simulink model "lift"  (R2015b)
settings: Solver=FixedStepAuto  StartTime=0.0  StopTime=200  FixedStep=1  MaxStep=10  RelTol=1e-3
libraries: simulink x8
settings Model: Creator=DNikolaev  LastModifiedBy=DNikolaev

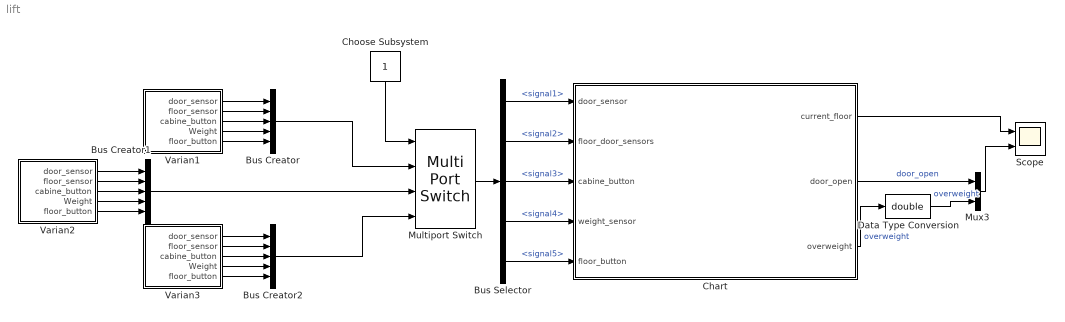
== system lift ==
  Bus Creator : BusCreator  Inputs=5
  Bus Creator1 : BusCreator  Inputs=5
  Bus Creator2 : BusCreator  Inputs=5
  Bus Selector : BusSelector  OutputSignals=signal1,signal2,signal3,signal4,signal5
  Chart : Stateflow chart  TreatAsAtomicUnit=on
  Choose Subsystem : Constant
  Data Type Conversion : DataTypeConversion  OutDataTypeStr=double
  Multiport Switch : MultiPortSwitch
  Mux3 : Mux  Inputs=2
  Scope : Scope  NumInputPorts=2
  Varian1 : Subsystem
  Varian2 : Subsystem
  Varian3 : Subsystem
  wires:
  Chart/1(current_floor) -> Scope/1
  Chart/2(door_open) -> Mux3/1  "door_open"
  Varian1/1(door_sensor) -> Bus Creator/1
  Varian1/2(floor_sensor) -> Bus Creator/2
  Varian1/3(cabine_button) -> Bus Creator/3
  Varian1/4(Weight) -> Bus Creator/4
  Varian1/5(floor_button) -> Bus Creator/5
  Multiport Switch/1 -> Bus Selector/1
  Bus Creator/1 -> Multiport Switch/2
  Bus Creator1/1 -> Multiport Switch/3
  Bus Creator2/1 -> Multiport Switch/4
  Choose Subsystem/1 -> Multiport Switch/1
  Varian3/1(door_sensor) -> Bus Creator2/1
  Varian3/2(floor_sensor) -> Bus Creator2/2
  Varian3/3(cabine_button) -> Bus Creator2/3
  Varian3/4(Weight) -> Bus Creator2/4
  Varian3/5(floor_button) -> Bus Creator2/5
  Chart/3(overweight) -> Data Type Conversion/1  "overweight"
  Mux3/1 -> Scope/2
  Varian2/3(cabine_button) -> Bus Creator1/3
  Varian2/2(floor_sensor) -> Bus Creator1/2
  Varian2/5(floor_button) -> Bus Creator1/5
  Varian2/4(Weight) -> Bus Creator1/4
  Varian2/1(door_sensor) -> Bus Creator1/1
  Bus Selector/5 -> Chart/5(floor_button)  "<signal5>"
  Bus Selector/4 -> Chart/4(weight_sensor)  "<signal4>"
  Bus Selector/2 -> Chart/2(floor_door_sensors)  "<signal2>"
  Bus Selector/1 -> Chart/1(door_sensor)  "<signal1>"
  Bus Selector/3 -> Chart/3(cabine_button)  "<signal3>"
  Data Type Conversion/1 -> Mux3/2  "overweight"

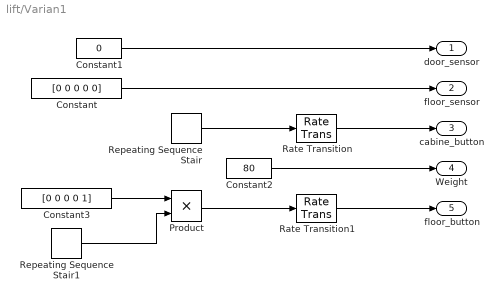
== system lift/Varian1 ==
  Constant : Constant  Value=[0 0 0 0 0]
  Constant1 : Constant  Value=0
  Constant2 : Constant  Value=80
  Constant3 : Constant  Value=[0 0 0 0 1]
  Product : Product
  Rate Transition : RateTransition  OutPortSampleTime=1
  Rate Transition1 : RateTransition  OutPortSampleTime=1
  Repeating Sequence Stair : simulink/Sources/Repeating Sequence Stair  OutValues=[0 0 0 0 0 0 0 0 0 2 0 0 0 0 0 0]  tsamp=10  OutMin=[]  OutMax=[]  OutDataTypeStr=double  OutputDataTypeScalingMode=double  OutDataType=fixdt(0,8)  ConRadixGroup=Best Precision: Vector-wise  OutScaling=2^-12
  Repeating Sequence Stair1 : simulink/Sources/Repeating Sequence Stair  OutValues=[0 0 1 0 0 0 0 0 0 0 0 0 0 0 0 0]  tsamp=10  OutMin=[]  OutMax=[]  OutDataTypeStr=double  OutputDataTypeScalingMode=double  OutDataType=fixdt(0,8)  ConRadixGroup=Best Precision: Vector-wise  OutScaling=2^-12
  door_sensor : Outport
  floor_sensor : Outport  Port=2
  cabine_button : Outport  Port=3
  Weight : Outport  Port=4
  floor_button : Outport  Port=5
  wires:
  Constant2/1 -> Weight/1
  Rate Transition/1 -> cabine_button/1
  Constant/1 -> floor_sensor/1
  Constant1/1 -> door_sensor/1
  Repeating Sequence Stair/1 -> Rate Transition/1
  Constant3/1 -> Product/1
  Rate Transition1/1 -> floor_button/1
  Repeating Sequence Stair1/1 -> Product/2
  Product/1 -> Rate Transition1/1

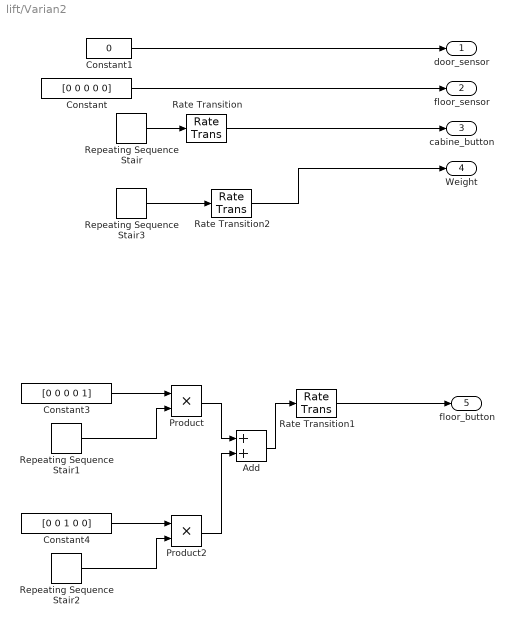
== system lift/Varian2 ==
  Add : Sum
  Constant : Constant  Value=[0 0 0 0 0]
  Constant1 : Constant  Value=0
  Constant3 : Constant  Value=[0 0 0 0 1]
  Constant4 : Constant  Value=[0 0 1 0 0]
  Product : Product
  Product2 : Product
  Rate Transition : RateTransition  OutPortSampleTime=1
  Rate Transition1 : RateTransition  OutPortSampleTime=1
  Rate Transition2 : RateTransition  OutPortSampleTime=1
  Repeating Sequence Stair : simulink/Sources/Repeating Sequence Stair  OutValues=[0 0 0 0 0 0 0 0 2 2 0 0 0 0 0 0]  tsamp=10  OutMin=[]  OutMax=[]  OutDataTypeStr=double  OutputDataTypeScalingMode=double  OutDataType=fixdt(0,8)  ConRadixGroup=Best Precision: Vector-wise  OutScaling=2^-12
  Repeating Sequence Stair1 : simulink/Sources/Repeating Sequence Stair  OutValues=[0 0 1 0 0 0 0 0 0 0 0 0 0 0 0 0]  tsamp=10  OutMin=[]  OutMax=[]  OutDataTypeStr=double  OutputDataTypeScalingMode=double  OutDataType=fixdt(0,8)  ConRadixGroup=Best Precision: Vector-wise  OutScaling=2^-12
  Repeating Sequence Stair2 : simulink/Sources/Repeating Sequence Stair  OutValues=[0 0 0 0 0 0 0 0 0 0 0 0 0 1 0]  tsamp=10  OutMin=[]  OutMax=[]  OutDataTypeStr=double  OutputDataTypeScalingMode=double  OutDataType=fixdt(0,8)  ConRadixGroup=Best Precision: Vector-wise  OutScaling=2^-12
  Repeating Sequence Stair3 : simulink/Sources/Repeating Sequence Stair  OutValues=[0 0 0 0 0 0 0 0 400 310 0 0 0 0 0 0]  tsamp=10  OutMin=[]  OutMax=[]  OutDataTypeStr=double  OutputDataTypeScalingMode=double  OutDataType=fixdt(0,8)  ConRadixGroup=Best Precision: Vector-wise  OutScaling=2^-12
  door_sensor : Outport
  floor_sensor : Outport  Port=2
  cabine_button : Outport  Port=3
  Weight : Outport  Port=4
  floor_button : Outport  Port=5
  wires:
  Product/1 -> Add/1
  Repeating Sequence Stair1/1 -> Product/2
  Rate Transition1/1 -> floor_button/1
  Constant3/1 -> Product/1
  Repeating Sequence Stair/1 -> Rate Transition/1
  Constant1/1 -> door_sensor/1
  Constant/1 -> floor_sensor/1
  Rate Transition/1 -> cabine_button/1
  Repeating Sequence Stair3/1 -> Rate Transition2/1
  Repeating Sequence Stair2/1 -> Product2/2
  Constant4/1 -> Product2/1
  Product2/1 -> Add/2
  Add/1 -> Rate Transition1/1
  Rate Transition2/1 -> Weight/1

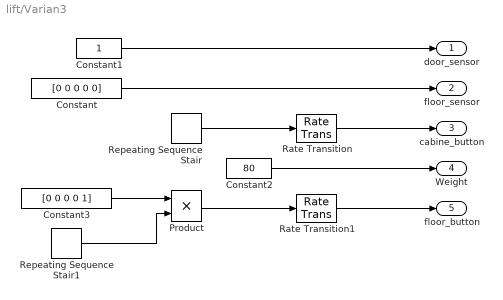
== system lift/Varian3 ==
  Constant : Constant  Value=[0 0 0 0 0]
  Constant1 : Constant
  Constant2 : Constant  Value=80
  Constant3 : Constant  Value=[0 0 0 0 1]
  Product : Product
  Rate Transition : RateTransition  OutPortSampleTime=1
  Rate Transition1 : RateTransition  OutPortSampleTime=1
  Repeating Sequence Stair : simulink/Sources/Repeating Sequence Stair  OutValues=[0 0 0 0 0 0 0 0 2 0 0 0 0 0 0 0]  tsamp=10  OutMin=[]  OutMax=[]  OutDataTypeStr=double  OutputDataTypeScalingMode=double  OutDataType=fixdt(0,8)  ConRadixGroup=Best Precision: Vector-wise  OutScaling=2^-12
  Repeating Sequence Stair1 : simulink/Sources/Repeating Sequence Stair  OutValues=[0 0 1 0 0 0 0 0 0 0 0 0 0 0 0 0]  tsamp=10  OutMin=[]  OutMax=[]  OutDataTypeStr=double  OutputDataTypeScalingMode=double  OutDataType=fixdt(0,8)  ConRadixGroup=Best Precision: Vector-wise  OutScaling=2^-12
  door_sensor : Outport
  floor_sensor : Outport  Port=2
  cabine_button : Outport  Port=3
  Weight : Outport  Port=4
  floor_button : Outport  Port=5
  wires:
  Constant2/1 -> Weight/1
  Rate Transition/1 -> cabine_button/1
  Constant/1 -> floor_sensor/1
  Constant1/1 -> door_sensor/1
  Repeating Sequence Stair/1 -> Rate Transition/1
  Constant3/1 -> Product/1
  Rate Transition1/1 -> floor_button/1
  Repeating Sequence Stair1/1 -> Product/2
  Product/1 -> Rate Transition1/1

== stateflow chart lift/Chart ==
  state Controller [parallel]
    du: [overweight,notenoughtweight]=weight(weight_sensor,max_weight,min_weight)
    settings: executionOrder=1
    state Idle
      en: status=1;
      open_cmd=0;
      close_cmd=0;
      move_to_cmd=0;
    state CalledFloor
      state CloseDoor3
        en:close_cmd=1;
        ex:close_cmd=0;
      state OpenDoor2
        en: open_cmd=1;
        ex: open_cmd=0;
      (junction 227) -> (junction 230) [order 1] : [floor_pressed_cmd(current_floor)~=0]
      (junction 230) -> CloseDoor3 [order 2] : after(3,sec)
      (junction 230) -> Controller.CalledFloor.OpenDoor2 [order 1] : [door_open==0]
      Controller.CalledFloor.OpenDoor2 -> CloseDoor3 : [door_open==1]
    state CalledCabine
      state OpenDoor2
        en: open_cmd=1;
        ex: open_cmd=0;
      state CloseDoor
        en:close_cmd=1;
      CloseDoor -> (junction 76)
      Controller.CalledCabine.OpenDoor2 -> (junction 76)
      (junction 76) -> CloseDoor [order 1] : [door_open==1&& overweight==0]
      (junction 76) -> Controller.CalledCabine.OpenDoor2 [order 3] : [door_open==0&& overweight==1]
    state Moving
      en: status=2;
      state Idle
      state MoveReady
        en: ready=1;
      state Move1floor
        en:current_floor=current_floor+sign(move_to_cmd-current_floor);
      state OpenDoor1
        en: open_cmd=1;
        ex: open_cmd=0;
      state CloseDoor2
        en:close_cmd=1;
        ex:close_cmd=0;
      (default) -> Controller.Moving.Idle : {ready=0;}
      Controller.Moving.Idle -> (junction 160)
      (junction 160) -> MoveReady [order 1] : [current_floor==move_to_cmd]
      (junction 167) -> (junction 160) [order 2]
      (junction 174) -> (junction 160) [order 2] : [door_open==0]
      (junction 160) -> (junction 165) [order 2] : [current_floor~=move_to_cmd]
      (junction 165) -> Move1floor : after(10,sec)
      Move1floor -> (junction 167)
      (junction 167) -> (junction 177) [order 1] : [floor_pressed_cmd(current_floor)~=0&&current_floor~=move_to_cmd]
      (junction 177) -> OpenDoor1 [order 1] : [door_open==0]
      (junction 177) -> CloseDoor2 [order 2] : [door_open==1]
      OpenDoor1 -> (junction 177)
      (junction 174) -> CloseDoor2 [order 1] : [door_open==1]
      CloseDoor2 -> (junction 174)
    state Ready
      en: status=3;
      ex: ready=0;
      state OpenDoor
        en: open_cmd=1;
        ex: open_cmd=0;
      state CloseDoor1
        en:close_cmd=1;
        ex:close_cmd=0;
      (junction 105) -> OpenDoor [order 1] : [door_open==0]
      (junction 105) -> CloseDoor1 [order 2] : [door_open==1]
      OpenDoor -> (junction 105)
      (junction 135) -> CloseDoor1 [order 1] : [door_open==1]
      CloseDoor1 -> (junction 135)
    (default) -> Controller.Idle : {current_floor=1;}
    Controller.Idle -> (junction 227) [order 1] : [~isempty(find(floor_pressed_cmd))]
    CalledCabine -> Controller.Idle : [move_to_cmd==0]
    Controller.Idle -> (junction 76) [order 2] : [button_pressed_cmd~=0]
    (junction 227) -> Moving [order 2] : [door_open==0 && overweight==0]
        | { move_to_cmd=moveto(floor_pressed_cmd)}
    (junction 76) -> Moving [order 2] : [door_open==0 && overweight==0 && notenoughtweight==0]
        | { move_to_cmd=button_pressed_cmd;}
    CloseDoor3 -> Moving : [door_open==0 && overweight==0]
        | { move_to_cmd=current_floor}
    Moving -> (junction 105) : [ready==1]
  state Doors [parallel]
    settings: executionOrder=2
    state Closed
      en: door_open=0;
      state Idle
      state OpenRequest
      (default) -> Doors.Closed.Idle
      Doors.Closed.Idle -> OpenRequest : [open_cmd==1]
    state Opened
      en: door_open=1;
      state Idle
      state CloseRequest
      CloseRequest -> Doors.Opened.Idle [order 1] : [after(30,sec)]
      Doors.Opened.Idle -> CloseRequest : [close_cmd==1]
      CloseRequest -> Doors.Opened.Idle [order 3] : [door_sensor==1]
    (default) -> Closed
    OpenRequest -> Doors.Opened.Idle : [after(2,sec)]
    CloseRequest -> Closed [order 2] : [after(2,sec)]
  state CabineButtons [parallel]
    settings: executionOrder=3
    state Idle
      en:button_pressed_cmd=0;
    state Pressed_and_Waiting
      en:button_pressed_cmd=cabine_button
      du:button_pressed_cmd=cabine_button
    state Pressed_and_Moving
      ex:button_pressed_cmd=0;
    (default) -> CabineButtons.Idle
    Pressed_and_Moving -> CabineButtons.Idle : [status==1']
    CabineButtons.Idle -> CabineButtons.Pressed_and_Waiting : [cabine_button>0]
    CabineButtons.Pressed_and_Waiting -> CabineButtons.Idle [order 2] : [after(20,sec)]
    CabineButtons.Pressed_and_Waiting -> Pressed_and_Moving [order 1] : [status==2]
  state FloorButtons [parallel]
    en: floor_pressed_cmd=[0 0 0 0 0];
    du:floor_pressed_cmd=[fb1,fb2,fb3,fb4,fb5];
    settings: executionOrder=4
    state FlooreButton1 [parallel]
      settings: executionOrder=1
      state Idle
        en:fb1=0;
      state Pressed_and_Waiting
        en:fb1=floor_button(1)
      (default) -> FloorButtons.FlooreButton1.Idle
      FloorButtons.FlooreButton1.Pressed_and_Waiting -> FloorButtons.FlooreButton1.Idle [order 1] : [current_floor==1 && door_open==1]
      FloorButtons.FlooreButton1.Idle -> FloorButtons.FlooreButton1.Pressed_and_Waiting : [floor_button(1)~=0]
      FloorButtons.FlooreButton1.Pressed_and_Waiting -> FloorButtons.FlooreButton1.Idle [order 2] : [after(200,sec)]
    state FlooreButton2 [parallel]
      settings: executionOrder=2
      state Idle
        en:fb2=0;
      state Pressed_and_Waiting
        en:fb2=floor_button(2)
      (default) -> FloorButtons.FlooreButton2.Idle
      FloorButtons.FlooreButton2.Pressed_and_Waiting -> FloorButtons.FlooreButton2.Idle [order 1] : [current_floor==2 && door_open==1]
      FloorButtons.FlooreButton2.Idle -> FloorButtons.FlooreButton2.Pressed_and_Waiting : [floor_button(2)~=0]
      FloorButtons.FlooreButton2.Pressed_and_Waiting -> FloorButtons.FlooreButton2.Idle [order 2] : [after(200,sec)]
    state FlooreButton3 [parallel]
      settings: executionOrder=3
      state Idle
        en:fb3=0;
      state Pressed_and_Waiting
        en:fb3=floor_button(3)
      (default) -> FloorButtons.FlooreButton3.Idle
      FloorButtons.FlooreButton3.Pressed_and_Waiting -> FloorButtons.FlooreButton3.Idle [order 1] : [current_floor==3 && door_open==1]
      FloorButtons.FlooreButton3.Idle -> FloorButtons.FlooreButton3.Pressed_and_Waiting : [floor_button(3)~=0]
      FloorButtons.FlooreButton3.Pressed_and_Waiting -> FloorButtons.FlooreButton3.Idle [order 2] : [after(200,sec)]
    state FlooreButton4 [parallel]
      settings: executionOrder=4
      state Idle
        en:fb4=0;
      state Pressed_and_Waiting
        en:fb4=floor_button(4)
      (default) -> FloorButtons.FlooreButton4.Idle
      FloorButtons.FlooreButton4.Pressed_and_Waiting -> FloorButtons.FlooreButton4.Idle [order 1] : [current_floor==4 && door_open==1]
      FloorButtons.FlooreButton4.Idle -> FloorButtons.FlooreButton4.Pressed_and_Waiting : [floor_button(4)~=0]
      FloorButtons.FlooreButton4.Pressed_and_Waiting -> FloorButtons.FlooreButton4.Idle [order 2] : [after(200,sec)]
    state FlooreButton5 [parallel]
      settings: executionOrder=5
      state Idle
        en:fb5=0;
      state Pressed_and_Waiting
        en:fb5=floor_button(5)
      (default) -> FloorButtons.FlooreButton5.Idle
      FloorButtons.FlooreButton5.Pressed_and_Waiting -> FloorButtons.FlooreButton5.Idle [order 1] : [current_floor==5 && door_open==1]
      FloorButtons.FlooreButton5.Idle -> FloorButtons.FlooreButton5.Pressed_and_Waiting : [floor_button(5)~=0]
      FloorButtons.FlooreButton5.Pressed_and_Waiting -> FloorButtons.FlooreButton5.Idle [order 2] : [after(200,sec)]
  (junction 135) -> Controller.Idle [order 2] : [door_open==0]
  data: weight_sens function_input; ov function_output; max function_input; min function_input; nev function_output; fpc function_input; move function_output; current_floor output; door_sensor input size=1; floor_door_sensors input size=5; cabine_button input; status local size=1; button_pressed_cmd local size=1; door_open output size=1; move_to_cmd local [1..5]; close_cmd local size=1; open_cmd local size=1; weight_sensor input size=1; max_weight constant double size=1 =320; min_weight constant double size=1 =20; overweight output; floor_button input; floor_pressed_cmd local; fb1 local; fb2 local; fb3 local; fb4 local; fb5 local; ready local; notenoughtweight local
  function [ov,nev] = weight(weight_sens,max,min):
    | function [ov,nev] = weight(weight_sens,max,min)
    | ov=(weight_sens>max);
    | nev=(weight_sens<min);
  function move=moveto(fpc):
    | function move=moveto(fpc)
    | move=1;
    | for i=5:-1:1
    |     if fpc(i)~=0
    |         move=i;
    |     end;
    | end;
